simulink model "EarDrumSimulator"  (R2024a)
settings: Solver=daessc  StartTime=0.0  StopTime=5  RelTol=1e-3
libraries: acoustic_lib x19, nesl_utility x4, simulink x1
settings Model: Creator=andychen  LastModifiedBy=jibrahim
settings DataIOCC: OutputOption=SpecifiedOutputTimes  OutputTimes=0:1/44100:5

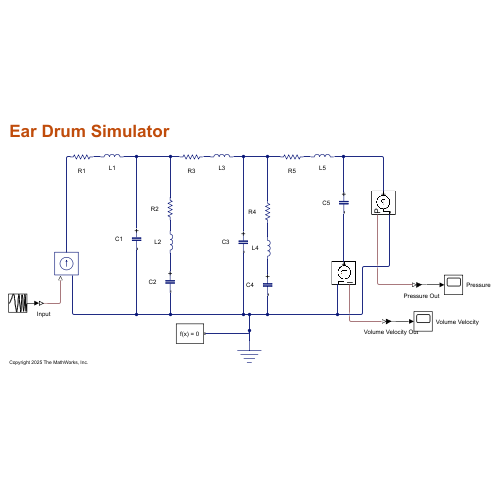
[thumbnail: Simulink's stored preview of the top-level diagram]
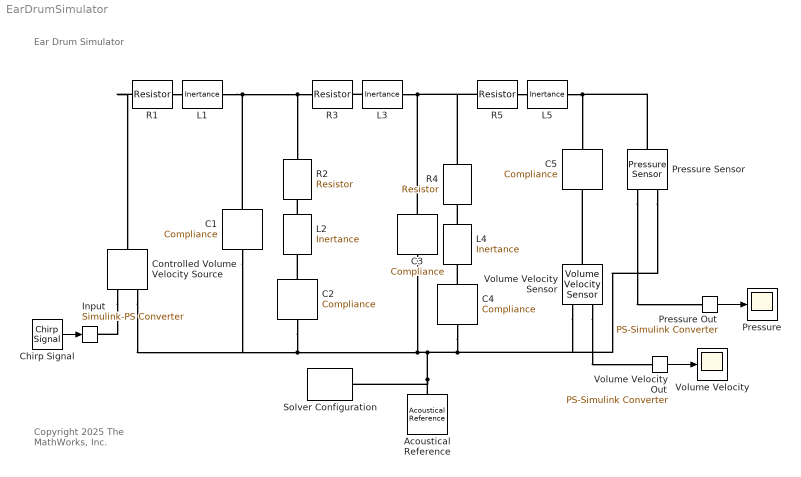
== system EarDrumSimulator ==
  note: Ear Drum Simulator
  note: Copyright 2025 The MathWorks, Inc.
  Acoustical Reference : acoustic_lib/Acoustical Elements/Acoustical Reference
      settings: SourceProductName=Acoustic  InternalSimscapePortConfiguration="{\"Bottom\":[],\"Left\":[{\"id\":\"pp\",\"label\":\"\",\"type\":\"acoustic.acoustic\"}],\"Right\":[],\"Top\":[]}"
  C1 : acoustic_lib/Acoustical Elements/Compliance  c=0.7e-12 m^3/Pa  r_c=0 Pa*s/m^3  g_c=0 m^3/(Pa*s)  u_specify=off  u_priority=None  u=0 m^3/s  u_nominal_specify=off  u_nominal_value=1  u_nominal_unit=m^3/s  p_specify=off  p_priority=None  p=0 Pa  p_nominal_specify=off  p_nominal_value=1  p_nominal_unit=Pa  Pc_specify=off  Pc_priority=High  Pc=0 Pa  Pc_nominal_specify=off  Pc_nominal_value=1  Pc_nominal_unit=Pa
      settings: SourceProductName=Acoustic  InternalSimscapePortConfiguration="{\"Bottom\":[],\"Left\":[{\"id\":\"pp\",\"label\":\"+\",\"type\":\"acoustic.acoustic\"}],\"Right\":[{\"id\":\"nn\",\"label\":\"-\",\"type\":\"acoustic.acoustic\"}],\"Top\":[]}"
  C2 : acoustic_lib/Acoustical Elements/Compliance  c=2.34e-12 m^3/Pa  r_c=0 Pa*s/m^3  g_c=0 m^3/(Pa*s)  u_specify=off  u_priority=None  u=0 m^3/s  u_nominal_specify=off  u_nominal_value=1  u_nominal_unit=m^3/s  p_specify=off  p_priority=None  p=0 Pa  p_nominal_specify=off  p_nominal_value=1  p_nominal_unit=Pa  Pc_specify=off  Pc_priority=High  Pc=0 Pa  Pc_nominal_specify=off  Pc_nominal_value=1  Pc_nominal_unit=Pa
      settings: SourceProductName=Acoustic  InternalSimscapePortConfiguration="{\"Bottom\":[],\"Left\":[{\"id\":\"pp\",\"label\":\"+\",\"type\":\"acoustic.acoustic\"}],\"Right\":[{\"id\":\"nn\",\"label\":\"-\",\"type\":\"acoustic.acoustic\"}],\"Top\":[]}"
  C3 : acoustic_lib/Acoustical Elements/Compliance  c=1.5e-12 m^3/Pa  r_c=0 Pa*s/m^3  g_c=0 m^3/(Pa*s)  u_specify=off  u_priority=None  u=0 m^3/s  u_nominal_specify=off  u_nominal_value=1  u_nominal_unit=m^3/s  p_specify=off  p_priority=None  p=0 Pa  p_nominal_specify=off  p_nominal_value=1  p_nominal_unit=Pa  Pc_specify=off  Pc_priority=High  Pc=0 Pa  Pc_nominal_specify=off  Pc_nominal_value=1  Pc_nominal_unit=Pa
      settings: SourceProductName=Acoustic  InternalSimscapePortConfiguration="{\"Bottom\":[],\"Left\":[{\"id\":\"pp\",\"label\":\"+\",\"type\":\"acoustic.acoustic\"}],\"Right\":[{\"id\":\"nn\",\"label\":\"-\",\"type\":\"acoustic.acoustic\"}],\"Top\":[]}"
  C4 : acoustic_lib/Acoustical Elements/Compliance  c=2.73e-12 m^3/Pa  r_c=0 Pa*s/m^3  g_c=0 m^3/(Pa*s)  u_specify=off  u_priority=None  u=0 m^3/s  u_nominal_specify=off  u_nominal_value=1  u_nominal_unit=m^3/s  p_specify=off  p_priority=None  p=0 Pa  p_nominal_specify=off  p_nominal_value=1  p_nominal_unit=Pa  Pc_specify=off  Pc_priority=High  Pc=0 Pa  Pc_nominal_specify=off  Pc_nominal_value=1  Pc_nominal_unit=Pa
      settings: SourceProductName=Acoustic  InternalSimscapePortConfiguration="{\"Bottom\":[],\"Left\":[{\"id\":\"pp\",\"label\":\"+\",\"type\":\"acoustic.acoustic\"}],\"Right\":[{\"id\":\"nn\",\"label\":\"-\",\"type\":\"acoustic.acoustic\"}],\"Top\":[]}"
  C5 : acoustic_lib/Acoustical Elements/Compliance  c=1.517e-12 m^3/Pa  r_c=0 Pa*s/m^3  g_c=0 m^3/(Pa*s)  u_specify=off  u_priority=None  u=0 m^3/s  u_nominal_specify=off  u_nominal_value=1  u_nominal_unit=m^3/s  p_specify=off  p_priority=None  p=0 Pa  p_nominal_specify=off  p_nominal_value=1  p_nominal_unit=Pa  Pc_specify=off  Pc_priority=High  Pc=0 Pa  Pc_nominal_specify=off  Pc_nominal_value=1  Pc_nominal_unit=Pa
      settings: SourceProductName=Acoustic  InternalSimscapePortConfiguration="{\"Bottom\":[],\"Left\":[{\"id\":\"pp\",\"label\":\"+\",\"type\":\"acoustic.acoustic\"}],\"Right\":[{\"id\":\"nn\",\"label\":\"-\",\"type\":\"acoustic.acoustic\"}],\"Top\":[]}"
  Chirp Signal : simulink/Sources/Chirp Signal  f1=10  T=5  f2=20e3
  Controlled Volume Velocity Source : acoustic_lib/Acoustical Sources/Controlled Volume Velocity Source
      settings: SourceProductName=Acoustic  InternalSimscapePortConfiguration="{\"Bottom\":[],\"Left\":[{\"id\":\"head\",\"label\":\"\",\"type\":\"acoustic.acoustic\"}],\"Right\":[{\"id\":\"uT\",\"label\":\"\",\"type\":\"input\"},{\"id\":\"tail\",\"label\":\"\",\"type\":\"acoustic.acoustic\"}],\"Top\":[]}"
  Input : nesl_utility/Simulink-PS Converter  PhysicalDomain=network_engine_domain  SubClassName=ps_input  LeftPortType=input  RightPortType=output  PseudoPeriodic=off  Frequencies=[]  NoiseDistribution=none  NoiseParameters=[]  Unit=1  AffineConversion=off  FilteringAndDerivatives=provide  SimscapeFilterOrder=1  InputFilterTimeConstant=0.001  UdotUserProvided=0
  L1 : acoustic_lib/Acoustical Elements/Inertance  m=82.9 Pa*s^2/m^3  r_m=1e-9 Pa*s/m^3  g_m=1e-9 m^3/(Pa*s)  u_specify=off  u_priority=None  u=0 m^3/s  u_nominal_specify=off  u_nominal_value=1  u_nominal_unit=m^3/s  p_specify=off  p_priority=None  p=0 Pa  p_nominal_specify=off  p_nominal_value=1  p_nominal_unit=Pa  U_m_specify=off  U_m_priority=High  U_m=0 m^3/s  U_m_nominal_specify=off  U_m_nominal_value=1  U_m_nominal_unit=m^3/s
      settings: SourceProductName=Acoustic  InternalSimscapePortConfiguration="{\"Bottom\":[],\"Left\":[{\"id\":\"pp\",\"label\":\"+\",\"type\":\"acoustic.acoustic\"}],\"Right\":[{\"id\":\"nn\",\"label\":\"-\",\"type\":\"acoustic.acoustic\"}],\"Top\":[]}"
  L2 : acoustic_lib/Acoustical Elements/Inertance  m=9400 Pa*s^2/m^3  r_m=1e-9 Pa*s/m^3  g_m=1e-9 m^3/(Pa*s)  u_specify=off  u_priority=None  u=0 m^3/s  u_nominal_specify=off  u_nominal_value=1  u_nominal_unit=m^3/s  p_specify=off  p_priority=None  p=0 Pa  p_nominal_specify=off  p_nominal_value=1  p_nominal_unit=Pa  U_m_specify=off  U_m_priority=High  U_m=0 m^3/s  U_m_nominal_specify=off  U_m_nominal_value=1  U_m_nominal_unit=m^3/s
      settings: SourceProductName=Acoustic  InternalSimscapePortConfiguration="{\"Bottom\":[],\"Left\":[{\"id\":\"pp\",\"label\":\"+\",\"type\":\"acoustic.acoustic\"}],\"Right\":[{\"id\":\"nn\",\"label\":\"-\",\"type\":\"acoustic.acoustic\"}],\"Top\":[]}"
  L3 : acoustic_lib/Acoustical Elements/Inertance  m=130.3 Pa*s^2/m^3  r_m=1e-9 Pa*s/m^3  g_m=1e-9 m^3/(Pa*s)  u_specify=off  u_priority=None  u=0 m^3/s  u_nominal_specify=off  u_nominal_value=1  u_nominal_unit=m^3/s  p_specify=off  p_priority=None  p=0 Pa  p_nominal_specify=off  p_nominal_value=1  p_nominal_unit=Pa  U_m_specify=off  U_m_priority=High  U_m=0 m^3/s  U_m_nominal_specify=off  U_m_nominal_value=1  U_m_nominal_unit=m^3/s
      settings: SourceProductName=Acoustic  InternalSimscapePortConfiguration="{\"Bottom\":[],\"Left\":[{\"id\":\"pp\",\"label\":\"+\",\"type\":\"acoustic.acoustic\"}],\"Right\":[{\"id\":\"nn\",\"label\":\"-\",\"type\":\"acoustic.acoustic\"}],\"Top\":[]}"
  L4 : acoustic_lib/Acoustical Elements/Inertance  m=983.8 Pa*s^2/m^3  r_m=1e-9 Pa*s/m^3  g_m=1e-9 m^3/(Pa*s)  u_specify=off  u_priority=None  u=0 m^3/s  u_nominal_specify=off  u_nominal_value=1  u_nominal_unit=m^3/s  p_specify=off  p_priority=None  p=0 Pa  p_nominal_specify=off  p_nominal_value=1  p_nominal_unit=Pa  U_m_specify=off  U_m_priority=High  U_m=0 m^3/s  U_m_nominal_specify=off  U_m_nominal_value=1  U_m_nominal_unit=m^3/s
      settings: SourceProductName=Acoustic  InternalSimscapePortConfiguration="{\"Bottom\":[],\"Left\":[{\"id\":\"pp\",\"label\":\"+\",\"type\":\"acoustic.acoustic\"}],\"Right\":[{\"id\":\"nn\",\"label\":\"-\",\"type\":\"acoustic.acoustic\"}],\"Top\":[]}"
  L5 : acoustic_lib/Acoustical Elements/Inertance  m=133.4 Pa*s^2/m^3  r_m=1e-9 Pa*s/m^3  g_m=1e-9 m^3/(Pa*s)  u_specify=off  u_priority=None  u=0 m^3/s  u_nominal_specify=off  u_nominal_value=1  u_nominal_unit=m^3/s  p_specify=off  p_priority=None  p=0 Pa  p_nominal_specify=off  p_nominal_value=1  p_nominal_unit=Pa  U_m_specify=off  U_m_priority=High  U_m=0 m^3/s  U_m_nominal_specify=off  U_m_nominal_value=1  U_m_nominal_unit=m^3/s
      settings: SourceProductName=Acoustic  InternalSimscapePortConfiguration="{\"Bottom\":[],\"Left\":[{\"id\":\"pp\",\"label\":\"+\",\"type\":\"acoustic.acoustic\"}],\"Right\":[{\"id\":\"nn\",\"label\":\"-\",\"type\":\"acoustic.acoustic\"}],\"Top\":[]}"
  Pressure : Scope
  Pressure Out : nesl_utility/PS-Simulink Converter  PhysicalDomain=network_engine_domain  SubClassName=ps_output  LeftPortType=input  RightPortType=output  PseudoPeriodic=off  Frequencies=[]  VectorFormat=inherit  Unit=inherit  AffineConversion=off
  Pressure Sensor : acoustic_lib/Acoustical Sensors/Pressure Sensor
      settings: SourceProductName=Acoustic  InternalSimscapePortConfiguration="{\"Bottom\":[],\"Left\":[{\"id\":\"pp\",\"label\":\"+\",\"type\":\"acoustic.acoustic\"}],\"Right\":[{\"id\":\"p\",\"label\":\"P\",\"type\":\"output\"},{\"id\":\"nn\",\"label\":\"-\",\"type\":\"acoustic.acoustic\"}],\"Top\":[]}"
  R1 : acoustic_lib/Acoustical Elements/Resistor  R_r=4.22e5 Pa*s/m^3  u_specify=off  u_priority=None  u=0 m^3/s  u_nominal_specify=off  u_nominal_value=1  u_nominal_unit=m^3/s  p_specify=off  p_priority=None  p=0 Pa  p_nominal_specify=off  p_nominal_value=1  p_nominal_unit=Pa
      settings: SourceProductName=Acoustic  InternalSimscapePortConfiguration="{\"Bottom\":[],\"Left\":[{\"id\":\"pp\",\"label\":\"+\",\"type\":\"acoustic.acoustic\"}],\"Right\":[{\"id\":\"nn\",\"label\":\"-\",\"type\":\"acoustic.acoustic\"}],\"Top\":[]}"
  R2 : acoustic_lib/Acoustical Elements/Resistor  R_r=55.66e6 Pa*s/m^3  u_specify=off  u_priority=None  u=0 m^3/s  u_nominal_specify=off  u_nominal_value=1  u_nominal_unit=m^3/s  p_specify=off  p_priority=None  p=0 Pa  p_nominal_specify=off  p_nominal_value=1  p_nominal_unit=Pa
      settings: SourceProductName=Acoustic  InternalSimscapePortConfiguration="{\"Bottom\":[],\"Left\":[{\"id\":\"pp\",\"label\":\"+\",\"type\":\"acoustic.acoustic\"}],\"Right\":[{\"id\":\"nn\",\"label\":\"-\",\"type\":\"acoustic.acoustic\"}],\"Top\":[]}"
  R3 : acoustic_lib/Acoustical Elements/Resistor  R_r=4.22e5 Pa*s/m^3  u_specify=off  u_priority=None  u=0 m^3/s  u_nominal_specify=off  u_nominal_value=1  u_nominal_unit=m^3/s  p_specify=off  p_priority=None  p=0 Pa  p_nominal_specify=off  p_nominal_value=1  p_nominal_unit=Pa
      settings: SourceProductName=Acoustic  InternalSimscapePortConfiguration="{\"Bottom\":[],\"Left\":[{\"id\":\"pp\",\"label\":\"+\",\"type\":\"acoustic.acoustic\"}],\"Right\":[{\"id\":\"nn\",\"label\":\"-\",\"type\":\"acoustic.acoustic\"}],\"Top\":[]}"
  R4 : acoustic_lib/Acoustical Elements/Resistor  R_r=27.99e6 Pa*s/m^3  u_specify=off  u_priority=None  u=0 m^3/s  u_nominal_specify=off  u_nominal_value=1  u_nominal_unit=m^3/s  p_specify=off  p_priority=None  p=0 Pa  p_nominal_specify=off  p_nominal_value=1  p_nominal_unit=Pa
      settings: SourceProductName=Acoustic  InternalSimscapePortConfiguration="{\"Bottom\":[],\"Left\":[{\"id\":\"pp\",\"label\":\"+\",\"type\":\"acoustic.acoustic\"}],\"Right\":[{\"id\":\"nn\",\"label\":\"-\",\"type\":\"acoustic.acoustic\"}],\"Top\":[]}"
  R5 : acoustic_lib/Acoustical Elements/Resistor  R_r=3.22e6 Pa*s/m^3  u_specify=off  u_priority=None  u=0 m^3/s  u_nominal_specify=off  u_nominal_value=1  u_nominal_unit=m^3/s  p_specify=off  p_priority=None  p=0 Pa  p_nominal_specify=off  p_nominal_value=1  p_nominal_unit=Pa
      settings: SourceProductName=Acoustic  InternalSimscapePortConfiguration="{\"Bottom\":[],\"Left\":[{\"id\":\"pp\",\"label\":\"+\",\"type\":\"acoustic.acoustic\"}],\"Right\":[{\"id\":\"nn\",\"label\":\"-\",\"type\":\"acoustic.acoustic\"}],\"Top\":[]}"
  Solver Configuration : nesl_utility/Solver Configuration  PhysicalDomain=network_engine_domain  SubClassName=solver  LeftPortType=input  RightPortType=generic  Tones=[]  Harmonics=[]  SimulateNoise=off  Profile=off  UseLocalSampling=off  EnableSwitchedLinearOptims=on  FrequencyDomain=off  UseCCode=off  RelTol=0.001  AbsTol=0.001  MinStep=1e-09  ToWorkspace=off  RevertToSquareIcSolve=off  NumHomotopyIterations=100  PhasorMode=off  PhasorModeNumHarmonics=1  ConsistencySolver=NEWTON_XTOL_AFTER_FTOL  IndexReductionMethod=DerivativeReplacement  DoDC=off  ResidualTolerance=1e-09  ConsistencyTolSource=GLOBAL  ConsistencyAbsTol=0.001  ConsistencyRelTol=0.001  ConsistencyTolFactor=0.001  UseLocalSolver=off  LocalSolverChoice=NE_BACKWARD_EULER_ADVANCER  ResolveIndetEquations=on  FunctionEvalNumThread=1  LocalSolverSampleTime=0.001  DoFixedCost=off  MaxNonlinIter=3  MaxModeIter=2  ComputeImpulses=off  ImpulseIterations=2  LinearAlgebra=auto  LinearAlgebraNumThread=0  EquationFormulation=NE_TIME_EF  DelaysMemoryBudget=1024  AutomaticFiltering=on  FilteringTimeConstant=0.001  PartitionStorageMethod=AS_NEEDED  PartitionMemoryBudget=1024  PartitionMethod=ROBUST  MultibodyUseLocalSolver=off  MultibodyLocalSolverChoice=ODE1  MultibodyLocalSolverSampleTime=0.001
  Volume Velocity : Scope
  Volume Velocity Sensor : acoustic_lib/Acoustical Sensors/Volume Velocity Sensor
      settings: SourceProductName=Acoustic  InternalSimscapePortConfiguration="{\"Bottom\":[],\"Left\":[{\"id\":\"pp\",\"label\":\"+\",\"type\":\"acoustic.acoustic\"}],\"Right\":[{\"id\":\"u\",\"label\":\"I\",\"type\":\"output\"},{\"id\":\"nn\",\"label\":\"-\",\"type\":\"acoustic.acoustic\"}],\"Top\":[]}"
  Volume Velocity Out : nesl_utility/PS-Simulink Converter  PhysicalDomain=network_engine_domain  SubClassName=ps_output  LeftPortType=input  RightPortType=output  PseudoPeriodic=off  Frequencies=[]  VectorFormat=inherit  Unit=inherit  AffineConversion=off
  wires:
  Volume Velocity Out/1 -> Volume Velocity/1
  Chirp Signal/1 -> Input/1
  Pressure Out/1 -> Pressure/1
  connections:
  C3/LConn1 -- R5/LConn1 -- R4/LConn1 -- L3/RConn1
  L2/LConn1 -- R2/RConn1
  C2/LConn1 -- L2/RConn1
  L4/LConn1 -- R4/RConn1
  C4/LConn1 -- L4/RConn1
  R5/RConn1 -- L5/LConn1
  C1/LConn1 -- L1/RConn1 -- R3/LConn1 -- R2/LConn1
  R1/RConn1 -- L1/LConn1
  L3/LConn1 -- R3/RConn1
  Acoustical Reference/LConn1 -- Solver Configuration/RConn1 -- Controlled Volume Velocity Source/RConn2 -- C1/RConn1 -- C2/RConn1 -- C3/RConn1 -- Volume Velocity Sensor/RConn2 -- Pressure Sensor/RConn2 -- C4/RConn1
  Controlled Volume Velocity Source/RConn1 -- Input/RConn1
  L5/RConn1 -- C5/LConn1 -- Pressure Sensor/LConn1
  Volume Velocity Sensor/LConn1 -- C5/RConn1
  R1/LConn1 -- Controlled Volume Velocity Source/LConn1
  Pressure Sensor/RConn1 -- Pressure Out/LConn1
  Volume Velocity Sensor/RConn1 -- Volume Velocity Out/LConn1
